simulink model "TapFilter"  (R2017a)
settings: Solver=VariableStepAuto  StartTime=0.0  StopTime=10.0  RelTol=1e-3
settings Model: Creator=Arthur  LastModifiedBy=Arthur

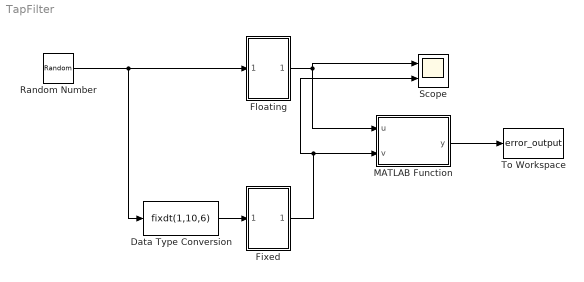
== system TapFilter ==
  Data Type Conversion : DataTypeConversion  OutDataTypeStr=fixdt(1,10,6)
  Fixed : Subsystem
  Floating : Subsystem
  MATLAB Function : MATLAB Function  TreatAsAtomicUnit=on
  Random Number : RandomNumber  SampleTime=0.1
  Scope : Scope  NumInputPorts=2
  To Workspace : ToWorkspace  VariableName=error_output  SaveFormat=Timeseries  SampleTime=-1
  wires:
  Floating/1(Out1) -> MATLAB Function/1(u), Scope/1
  Fixed/1(Out1) -> MATLAB Function/2(v), Scope/2
  MATLAB Function/1(y) -> To Workspace/1
  Random Number/1 -> Data Type Conversion/1, Floating/1(In1)
  Data Type Conversion/1 -> Fixed/1(In1)

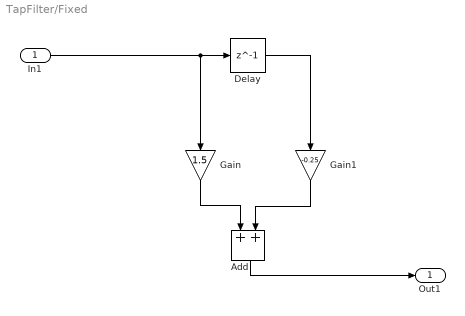
== system TapFilter/Fixed ==
  In1 : Inport
  Add : Sum  OutDataTypeStr=fixdt(1,10,6)
  Delay : Delay  DelayLength=1
  Gain : Gain  Gain=1.5  ParamDataTypeStr=fixdt(0,2,1)  OutDataTypeStr=fixdt(1,10,6)
  Gain1 : Gain  Gain=-0.25  ParamDataTypeStr=fixdt(1,3,2)  OutDataTypeStr=fixdt(1,10,6)
  Out1 : Outport
  wires:
  Add/1 -> Out1/1
  In1/1 -> Gain/1, Delay/1
  Gain/1 -> Add/1
  Gain1/1 -> Add/2
  Delay/1 -> Gain1/1

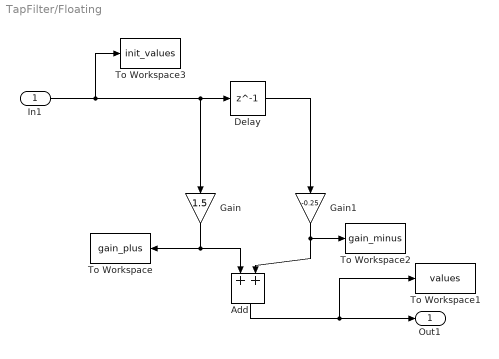
== system TapFilter/Floating ==
  In1 : Inport
  Add : Sum  OutDataTypeStr=double
  Delay : Delay  DelayLength=1
  Gain : Gain  Gain=1.5  ParamDataTypeStr=double  OutDataTypeStr=double
  Gain1 : Gain  Gain=-0.25  ParamDataTypeStr=double  OutDataTypeStr=double
  To Workspace : ToWorkspace  VariableName=gain_plus  SaveFormat=Timeseries  SampleTime=-1
  To Workspace1 : ToWorkspace  VariableName=values  SaveFormat=Timeseries  SampleTime=-1
  To Workspace2 : ToWorkspace  VariableName=gain_minus  SaveFormat=Timeseries  SampleTime=-1
  To Workspace3 : ToWorkspace  VariableName=init_values  SaveFormat=Timeseries  SampleTime=-1
  Out1 : Outport
  wires:
  Add/1 -> To Workspace1/1, Out1/1
  In1/1 -> To Workspace3/1, Gain/1, Delay/1
  Gain/1 -> To Workspace/1, Add/1
  Gain1/1 -> Add/2, To Workspace2/1
  Delay/1 -> Gain1/1

== matlab function TapFilter/MATLAB Function ==
  data: u input; y output; v input
function y = fcn(u,v)

u = double (u);
v = double (v);

y = abs(u - v);
